simulink model "IEEE13NF_unbal"  (Simulink 8.5)
settings: Solver=ode4  StartTime=0.0  StopTime=10  FixedStep=Ts  RelTol=1e-3
PreLoadFcn:
  | Ts=0.01;
PostLoadFcn:
  | Ts=0.01;
InitFcn:
  | Ts=0.01;
StartFcn:
  | Ts=0.01;
libraries: dspindex x6, opal_lib x2, rtlab x2, rtlab_phasor x1
settings Model: Creator=ZhiqiZhao  LastModifiedBy=Jaimie.Swartz
settings DebuggingCC: SolverPrmCheckMsg=warning  FcnCallInpInsideContextMsg=EnableAllAsWarning

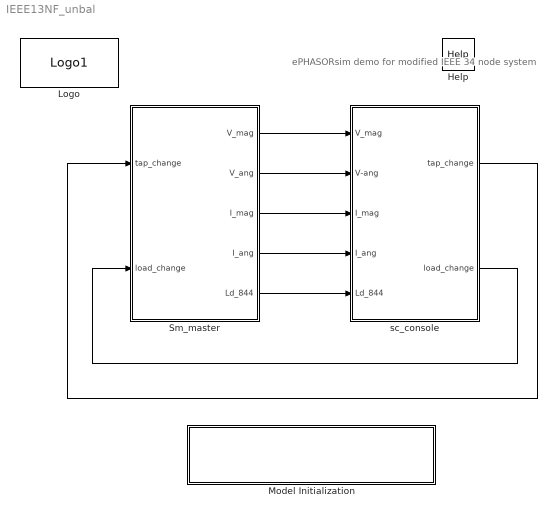
== system IEEE13NF_unbal ==
  note: ePHASORsim demo for
      | modified IEEE 34 node system
  Help : opal_lib/Help  docfile=../help/ePH_IEEE34.html
  Logo : opal_lib/Logo1  vide=[]
  Model Initialization : Subsystem  mask(Model Functions){InitFcnX=Ts=0.01;, prel=on, posl=on, inif=on, strf=on}
      mask prompts: InitFcnX "Initialisation"; prel "Preload Function"; posl "PostLoad Function"; inif "InitFcn"; strf "StartFcn"
      mask init:
      | currentBlock = gcb;
      | root = bdroot(currentBlock);
      | 
      | if ~strcmp(get_param(root,'BlockDiagramType'),'library')
      |     if prel==1
      |         set_param(root, 'PreLoadFcn', InitFcnX);
      |     else
      |         set_param(root, 'PreLoadFcn', '');
      |     end
      |     if inif==1
      |         set_param(root, 'InitFcn', InitFcnX);
      |     else
      |         set_param(root, 'InitFcn', '');
      |     end
      |     if strf==1
      |         set_param(root, 'StartFcn', InitFcnX);
      |     else
      |         set_param(root, 'StartFcn', '');
      |     end
      |     if posl==1
      |         set_param(root, 'PostLoadFcn', InitFcnX);
      |     else
      |         set_param(root, 'PostLoadFcn', '');
      |     end
      | end
      | 
      | pos = get_param(currentBlock, 'Position');
      | width = pos(3) - pos(1); height = pos(4) - pos(2);
      | txt = [ upper(root) '\n' '- InitFcn. . . . . '  get_param(root, 'InitFcn') ];
      settings: CopyFcn=set_param(gcb,'LinkStatus','none')
      mask Display: text(5, height*0.5, txt, 'horizontalAlignment', 'left', 'verticalAlignment', 'middle') ;
  Sm_master : Subsystem
  sc_console : Subsystem
  wires:
  Sm_master/1(V_mag) -> sc_console/1(V_mag)
  Sm_master/2(V_ang) -> sc_console/2(V-ang)
  Sm_master/5(Ld_844) -> sc_console/5(Ld_844)
  sc_console/1(tap_change) -> Sm_master/1(tap_change)
  sc_console/2(load_change) -> Sm_master/2(load_change)
  Sm_master/3(I_mag) -> sc_console/3(I_mag)
  Sm_master/4(I_ang) -> sc_console/4(I_ang)

== system IEEE13NF_unbal/Model Initialization ==

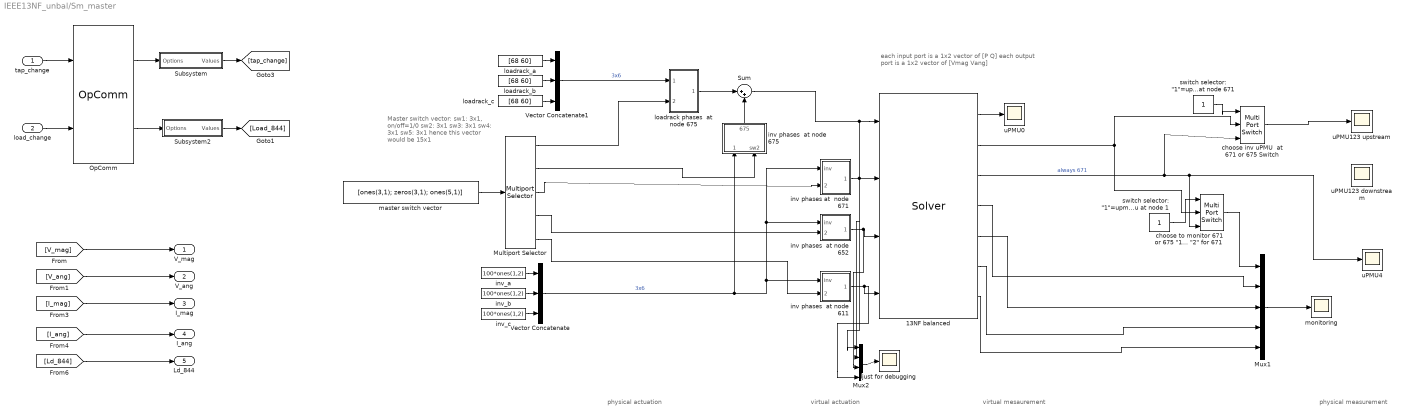
== system IEEE13NF_unbal/Sm_master ==
  note: Master switch vector:
      | sw1: 3x1, on/off=1/0
      | sw2: 3x1
      | sw3: 3x1
      | sw4: 3x1
      | sw5: 3x1
      | hence this vector would be 15x1
  note: virtual actuation
  note: virtual mesaurement
  note: physical measurement
  note: physical actuation
  note: each input port is a 1x2 vector of [P Q]
      | each output port is a 1x2 vector of [Vmag Vang]
  tap_change : Inport
  load_change : Inport  Port=2
  13NF balanced : rtlab_phasor/Solver  epname=System  extension=Excel  xls='IEEE13NF_unbal.xls'  raw='4992b.raw'  dyr='4992b.dyr'  cyme='ieee13.sxst'  powerfactory='network.dgs'  builtin=on  cyme_pf=''  cyme_unbalanced=on  lazy_netlist=on  capidir='CAPI'  fmudir='FMU'  capiprefix=capicomp_  fmuprefix=fmucomp_  logging=off  sim_mode=Dynamic simulation only (without power-flow)  pf_max_it=100  pf_tol_v=0.00000001  pf_flat_start=off  pf_smart_start=off  pf_export=on  np=1  exporty=off  dt=Ts  optim_threads=off  perflog_on=off  script_activate_postinit=off  script_postinit_name='python_integration_13NFunbal.py'
  Multiport Selector : dspindex/Multiport Selector  rowsOrCols=Rows  idxCellArray={ [1:3], [4:6], [7:9], 10,11 }  idxErrMode=Clip Index
  Mux1 : Mux  Inputs=5
  Mux2 : Mux
  OpComm : rtlab/OpComm  nbport=2  groupe_acq=1  subsys_rate=0  st=0  Synchronization=on  Interpolation=on  Threshold=1.0  Missed_Data=off  Sim_Time=off  Samples=off  dynSigOut=off  from_console=1  warning_done=off  writeOpCommFile=off  Offset=off
  Subsystem : Subsystem
  Subsystem2 : Subsystem
  Sum : Sum  Inputs=|++
  Vector Concatenate : Concatenate  NumInputs=3  Mode=Multidimensional array  ConcatenateDimension=2
  Vector Concatenate1 : Concatenate  NumInputs=3  Mode=Multidimensional array  ConcatenateDimension=2
  choose inv uPMU  at 671 or 675 Switch : MultiPortSwitch  Inputs=2
  "choose to monitor 671 or 675 \"1\" for 675 \"2\" for 671" : MultiPortSwitch  Inputs=2
  inv phases  at node 675 : Subsystem
  inv phases  at node 611 : Subsystem
  inv phases  at node 652 : Subsystem
  inv phases at  node 671 : Subsystem
  inv_a : Constant  Value=100*ones(1,2)
  inv_b : Constant  Value=100*ones(1,2)
  inv_c : Constant  Value=100*ones(1,2)
  just for debugging : Scope
      settings: SaveName=ScopeData30
  loadrack phases  at node 675 : Subsystem
  loadrack_a : Constant  Value=[68 60]
  loadrack_b : Constant  Value=[68 60]
  loadrack_c : Constant  Value=[68 60]
  master switch vector : Constant  Value=[ones(3,1); zeros(3,1); ones(5,1)]
  monitoring : Scope
      settings: SaveName=ScopeData31
  "switch selector: \"1\"=upmu at node 675 \"2\"=upmu at node 1" : Constant
  "switch selector: \"1\"=upmu at node 675 \"2\"=upmu at node 671" : Constant
  uPMU0 : Scope
  uPMU123 downstream : Scope
      settings: SaveName=ScopeData32
  uPMU123 upstream : Scope
      settings: SaveName=ScopeData33
  uPMU4 : Scope
      settings: SaveName=ScopeData34
  V_mag : Outport
  V_ang : Outport  Port=2
  I_mag : Outport  Port=3
  I_ang : Outport  Port=4
  Ld_844 : Outport  Port=5
  wires:
  tap_change/1 -> OpComm/1
  load_change/1 -> OpComm/2
  [V_mag] -> V_mag/1
  [V_ang] -> V_ang/1
  [I_ang] -> I_ang/1
  [I_mag] -> I_mag/1
  [Ld_844] -> Ld_844/1
  OpComm/1 -> Subsystem/1(Options)
  OpComm/2 -> Subsystem2/1(Options)
  Subsystem/1(Values) -> [tap_change]
  Subsystem2/1(Values) -> [Load_844]
  loadrack_a/1 -> Vector Concatenate1/1
  loadrack_b/1 -> Vector Concatenate1/2
  loadrack_c/1 -> Vector Concatenate1/3
  Vector Concatenate1/1 -> loadrack phases  at node 675/1(loadrack)  "3x6"
  inv_a/1 -> Vector Concatenate/1
  inv_b/1 -> Vector Concatenate/2
  inv_c/1 -> Vector Concatenate/3
  Sum/1 -> Mux2/1, 13NF balanced/1
  Vector Concatenate/1 -> inv phases  at node 675/1(loadrack), inv phases  at node 611/1(inv), inv phases at  node 671/1(inv), inv phases  at node 652/1(inv)  "3x6"
  inv phases at  node 671/1(671) -> Mux2/2, 13NF balanced/2
  inv phases  at node 652/1(652) -> 13NF balanced/3, Mux2/3
  inv phases  at node 611/1(611) -> 13NF balanced/4, Mux2/4
  13NF balanced/7 -> Mux1/5
  13NF balanced/5 -> Mux1/3
  13NF balanced/4 -> Mux1/2
  "switch selector: \"1\"=upmu at node 675 \"2\"=upmu at node 671"/1 -> choose inv uPMU  at 671 or 675 Switch/1
  13NF balanced/1 -> uPMU0/1
  choose inv uPMU  at 671 or 675 Switch/1 -> uPMU123 upstream/1
  13NF balanced/3 -> choose inv uPMU  at 671 or 675 Switch/3, "choose to monitor 671 or 675 \"1\" for 675 \"2\" for 671"/3, uPMU4/1  "always 671"
  "choose to monitor 671 or 675 \"1\" for 675 \"2\" for 671"/1 -> Mux1/1
  13NF balanced/6 -> Mux1/4
  Mux1/1 -> monitoring/1
  ? -> uPMU123 downstream/1
  loadrack phases  at node 675/1(675) -> Sum/1
  inv phases  at node 675/1(675) -> Sum/2
  master switch vector/1 -> Multiport Selector/1
  Multiport Selector/1 -> loadrack phases  at node 675/2(sw1)
  Multiport Selector/2 -> inv phases  at node 675/2(sw2)
  Multiport Selector/3 -> inv phases at  node 671/2(sw3)
  Multiport Selector/4 -> inv phases  at node 652/2(sw4)
  Multiport Selector/5 -> inv phases  at node 611/2(sw5)
  Mux2/1 -> just for debugging/1
  "switch selector: \"1\"=upmu at node 675 \"2\"=upmu at node 1"/1 -> "choose to monitor 671 or 675 \"1\" for 675 \"2\" for 671"/1
  13NF balanced/2 -> "choose to monitor 671 or 675 \"1\" for 675 \"2\" for 671"/2, choose inv uPMU  at 671 or 675 Switch/2

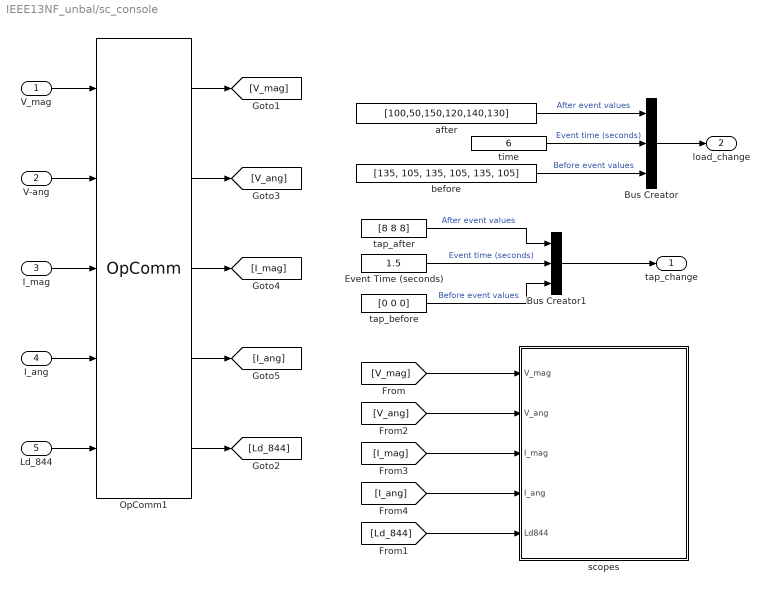
== system IEEE13NF_unbal/sc_console ==
  V_mag : Inport
  V-ang : Inport  Port=2
  I_mag : Inport  Port=3
  I_ang : Inport  Port=4
  Ld_844 : Inport  Port=5
  Bus Creator : BusCreator  Inputs=3
  Bus Creator1 : BusCreator  Inputs=3
  Event Time (seconds) : Constant  Value=1.5
  OpComm1 : rtlab/OpComm  nbport=5  groupe_acq=1  subsys_rate=0  st=0  Synchronization=on  Interpolation=on  Threshold=1.0  Missed_Data=off  Sim_Time=off  Samples=off  dynSigOut=off  from_console=0  warning_done=off  writeOpCommFile=off  Offset=off
  after : Constant  Value=[100,50,150,120,140,130]
  before : Constant  Value=[135, 105, 135, 105, 135, 105]
  scopes : Subsystem
  tap_after : Constant  Value=[8 8 8]
  tap_before : Constant  Value=[0 0 0]
  time : Constant  Value=6
  tap_change : Outport
  load_change : Outport  Port=2
  wires:
  V-ang/1 -> OpComm1/2
  V_mag/1 -> OpComm1/1
  OpComm1/1 -> [V_mag]
  OpComm1/2 -> [V_ang]
  time/1 -> Bus Creator/2  "Event time (seconds)"
  Bus Creator/1 -> load_change/1
  tap_after/1 -> Bus Creator1/1  "After event values"
  tap_before/1 -> Bus Creator1/3  "Before event values"
  Event Time (seconds)/1 -> Bus Creator1/2  "Event time (seconds)"
  Bus Creator1/1 -> tap_change/1
  after/1 -> Bus Creator/1  "After event values"
  before/1 -> Bus Creator/3  "Before event values"
  OpComm1/5 -> [Ld_844]
  Ld_844/1 -> OpComm1/5
  I_mag/1 -> OpComm1/3
  I_ang/1 -> OpComm1/4
  OpComm1/4 -> [I_ang]
  OpComm1/3 -> [I_mag]
  [V_mag] -> scopes/1(V_mag)
  [V_ang] -> scopes/2(V_ang)
  [I_mag] -> scopes/3(I_mag)
  [I_ang] -> scopes/4(I_ang)
  [Ld_844] -> scopes/5(Ld844)

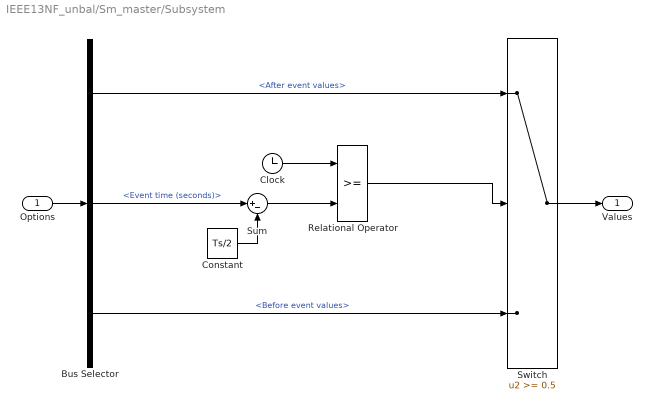
== system IEEE13NF_unbal/Sm_master/Subsystem ==
  Options : Inport
  Bus Selector : BusSelector  OutputSignals=After event values,Event time (seconds),Before event values
  Clock : Clock
  Constant : Constant  Value=Ts/2
  Relational Operator : RelationalOperator  OutDataTypeStr=boolean
  Sum : Sum  Inputs=|+-
  Switch : Switch  Threshold=0.5
  Values : Outport
  wires:
  Clock/1 -> Relational Operator/1
  Constant/1 -> Sum/2
  Sum/1 -> Relational Operator/2
  Bus Selector/2 -> Sum/1  "<Event time (seconds)>"
  Relational Operator/1 -> Switch/2
  Bus Selector/3 -> Switch/3  "<Before event values>"
  Bus Selector/1 -> Switch/1  "<After event values>"
  Switch/1 -> Values/1
  Options/1 -> Bus Selector/1

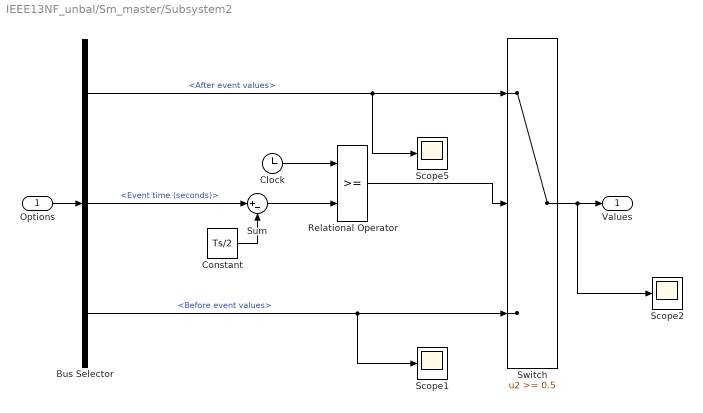
== system IEEE13NF_unbal/Sm_master/Subsystem2 ==
  Options : Inport
  Bus Selector : BusSelector  OutputSignals=After event values,Event time (seconds),Before event values
  Clock : Clock
  Constant : Constant  Value=Ts/2
  Relational Operator : RelationalOperator  OutDataTypeStr=boolean
  Scope1 : Scope
      settings: SaveName=ScopeData14
  Scope2 : Scope
      settings: SaveName=ScopeData15
  Scope5 : Scope
      settings: SaveName=ScopeData13
  Sum : Sum  Inputs=|+-
  Switch : Switch  Threshold=0.5
  Values : Outport
  wires:
  Clock/1 -> Relational Operator/1
  Constant/1 -> Sum/2
  Sum/1 -> Relational Operator/2
  Bus Selector/2 -> Sum/1  "<Event time (seconds)>"
  Relational Operator/1 -> Switch/2
  Bus Selector/3 -> Switch/3, Scope1/1  "<Before event values>"
  Bus Selector/1 -> Switch/1, Scope5/1  "<After event values>"
  Switch/1 -> Values/1, Scope2/1
  Options/1 -> Bus Selector/1

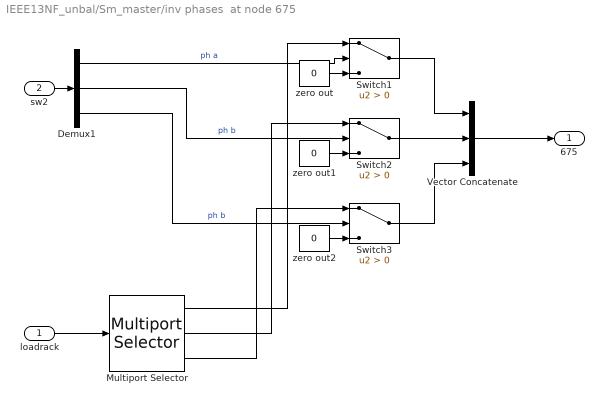
== system IEEE13NF_unbal/Sm_master/inv phases  at node 675 ==
  loadrack : Inport
  sw2 : Inport  Port=2
  Demux1 : Demux  Outputs=3
  Multiport Selector : dspindex/Multiport Selector  rowsOrCols=Columns  idxCellArray={ 1, 2, 3 }  idxErrMode=Clip Index
  Switch1 : Switch  Criteria=u2 > Threshold
  Switch2 : Switch  Criteria=u2 > Threshold
  Switch3 : Switch  Criteria=u2 > Threshold
  Vector Concatenate : Concatenate  NumInputs=3  ConcatenateDimension=2
  zero out : Constant  Value=0
  zero out1 : Constant  Value=0
  zero out2 : Constant  Value=0
  675 : Outport
  wires:
  Demux1/3 -> Switch3/2  "ph b"
  zero out2/1 -> Switch3/3
  Demux1/1 -> Switch1/2  "ph a"
  zero out/1 -> Switch1/3
  loadrack/1 -> Multiport Selector/1
  Switch2/1 -> Vector Concatenate/2
  Switch1/1 -> Vector Concatenate/1
  Switch3/1 -> Vector Concatenate/3
  Vector Concatenate/1 -> 675/1
  Multiport Selector/2 -> Switch2/1
  Multiport Selector/1 -> Switch1/1
  Multiport Selector/3 -> Switch3/1
  Demux1/2 -> Switch2/2  "ph b"
  zero out1/1 -> Switch2/3
  sw2/1 -> Demux1/1

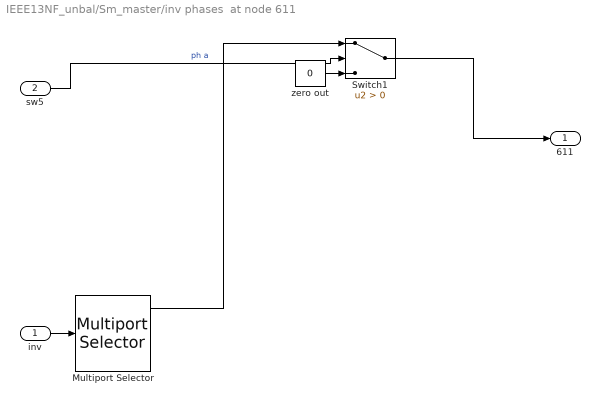
== system IEEE13NF_unbal/Sm_master/inv phases  at node 611 ==
  inv : Inport
  sw5 : Inport  Port=2
  Multiport Selector : dspindex/Multiport Selector  rowsOrCols=Columns  idxCellArray={ 1, 2, 3 }  idxErrMode=Clip Index
  Switch1 : Switch  Criteria=u2 > Threshold
  zero out : Constant  Value=0
  611 : Outport
  wires:
  sw5/1 -> Switch1/2  "ph a"
  zero out/1 -> Switch1/3
  Switch1/1 -> 611/1
  inv/1 -> Multiport Selector/1
  Multiport Selector/1 -> Switch1/1

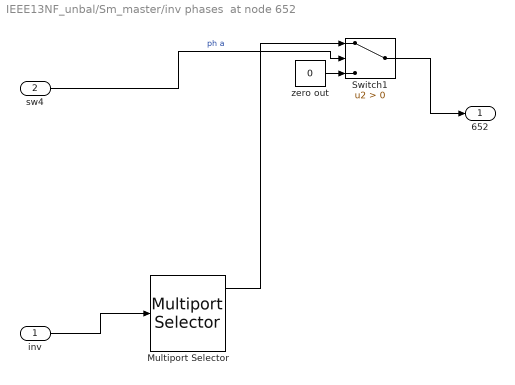
== system IEEE13NF_unbal/Sm_master/inv phases  at node 652 ==
  inv : Inport
  sw4 : Inport  Port=2
  Multiport Selector : dspindex/Multiport Selector  rowsOrCols=Columns  idxCellArray={ 1, 2, 3 }  idxErrMode=Clip Index
  Switch1 : Switch  Criteria=u2 > Threshold
  zero out : Constant  Value=0
  652 : Outport
  wires:
  sw4/1 -> Switch1/2  "ph a"
  zero out/1 -> Switch1/3
  Switch1/1 -> 652/1
  inv/1 -> Multiport Selector/1
  Multiport Selector/1 -> Switch1/1

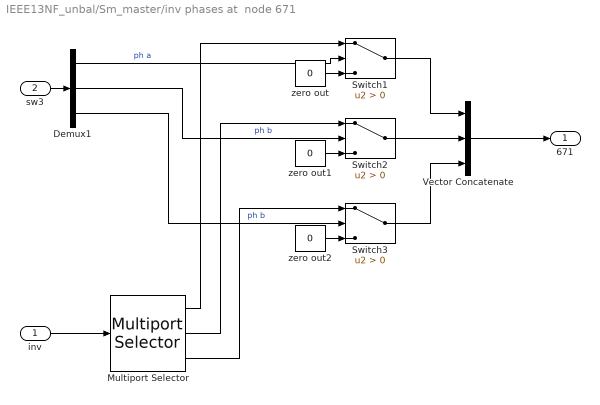
== system IEEE13NF_unbal/Sm_master/inv phases at  node 671 ==
  inv : Inport
  sw3 : Inport  Port=2
  Demux1 : Demux  Outputs=3
  Multiport Selector : dspindex/Multiport Selector  rowsOrCols=Columns  idxCellArray={ 1, 2, 3 }  idxErrMode=Clip Index
  Switch1 : Switch  Criteria=u2 > Threshold
  Switch2 : Switch  Criteria=u2 > Threshold
  Switch3 : Switch  Criteria=u2 > Threshold
  Vector Concatenate : Concatenate  NumInputs=3  ConcatenateDimension=2
  zero out : Constant  Value=0
  zero out1 : Constant  Value=0
  zero out2 : Constant  Value=0
  671 : Outport
  wires:
  Demux1/3 -> Switch3/2  "ph b"
  zero out2/1 -> Switch3/3
  Demux1/1 -> Switch1/2  "ph a"
  zero out/1 -> Switch1/3
  inv/1 -> Multiport Selector/1
  Switch2/1 -> Vector Concatenate/2
  Switch1/1 -> Vector Concatenate/1
  Switch3/1 -> Vector Concatenate/3
  Vector Concatenate/1 -> 671/1
  Multiport Selector/2 -> Switch2/1
  Multiport Selector/1 -> Switch1/1
  Multiport Selector/3 -> Switch3/1
  Demux1/2 -> Switch2/2  "ph b"
  zero out1/1 -> Switch2/3
  sw3/1 -> Demux1/1

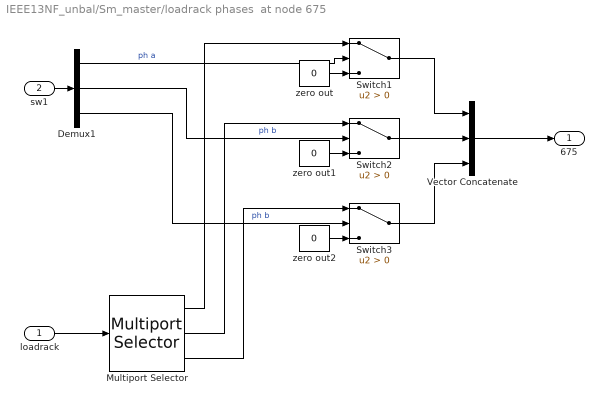
== system IEEE13NF_unbal/Sm_master/loadrack phases  at node 675 ==
  loadrack : Inport
  sw1 : Inport  Port=2
  Demux1 : Demux  Outputs=3
  Multiport Selector : dspindex/Multiport Selector  rowsOrCols=Columns  idxCellArray={ 1, 2, 3 }  idxErrMode=Clip Index
  Switch1 : Switch  Criteria=u2 > Threshold
  Switch2 : Switch  Criteria=u2 > Threshold
  Switch3 : Switch  Criteria=u2 > Threshold
  Vector Concatenate : Concatenate  NumInputs=3  ConcatenateDimension=2
  zero out : Constant  Value=0
  zero out1 : Constant  Value=0
  zero out2 : Constant  Value=0
  675 : Outport
  wires:
  Demux1/3 -> Switch3/2  "ph b"
  zero out2/1 -> Switch3/3
  Demux1/1 -> Switch1/2  "ph a"
  zero out/1 -> Switch1/3
  loadrack/1 -> Multiport Selector/1
  Switch2/1 -> Vector Concatenate/2
  Switch1/1 -> Vector Concatenate/1
  Switch3/1 -> Vector Concatenate/3
  Vector Concatenate/1 -> 675/1
  Multiport Selector/2 -> Switch2/1
  Multiport Selector/1 -> Switch1/1
  Multiport Selector/3 -> Switch3/1
  Demux1/2 -> Switch2/2  "ph b"
  zero out1/1 -> Switch2/3
  sw1/1 -> Demux1/1

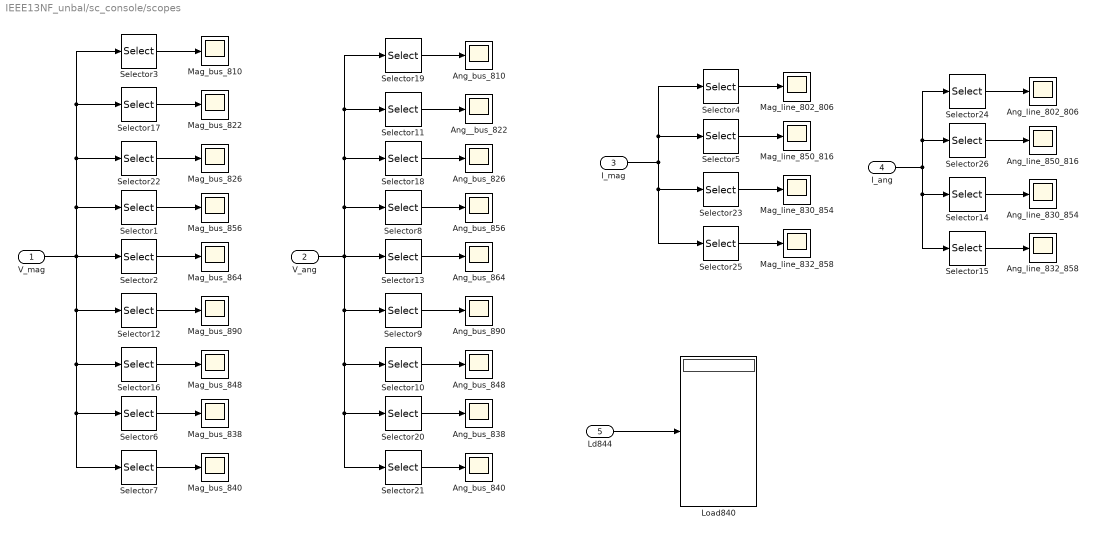
== system IEEE13NF_unbal/sc_console/scopes ==
  V_mag : Inport
  V_ang : Inport  Port=2
  I_mag : Inport  Port=3
  I_ang : Inport  Port=4
  Ld844 : Inport  Port=5
  Ang__bus_822 : Scope
      settings: YMin=0.92  YMax=1.07  SaveName=ScopeData8
  Ang_bus_{810,826,838,840,848,856,864,890} (8 alike) : Scope
      Ang_bus_810 settings: YMin=0.92  YMax=1.07  SaveName=ScopeData18
      Ang_bus_826 settings: YMin=0.92  YMax=1.07  SaveName=ScopeData9
      Ang_bus_838 settings: YMin=0.92  YMax=1.07  SaveName=ScopeData22
      Ang_bus_840 settings: YMin=0.92  YMax=1.07  SaveName=ScopeData25
      Ang_bus_848 settings: YMin=0.92  YMax=1.07  SaveName=ScopeData24
      Ang_bus_856 settings: YMin=0.92  YMax=1.07  SaveName=ScopeData10
      Ang_bus_864 settings: YMin=0.92  YMax=1.07  SaveName=ScopeData11
      Ang_bus_890 settings: YMin=0.92  YMax=1.07  SaveName=ScopeData23
  Ang_line_802_806 : Scope
      settings: YMin=0.92  YMax=1.07
  Ang_line_830_854 : Scope
      settings: YMin=0.92  YMax=1.07  SaveName=ScopeData20
  Ang_line_832_858 : Scope
      settings: YMin=0.92  YMax=1.07  SaveName=ScopeData27
  Ang_line_850_816 : Scope
      settings: YMin=0.92  YMax=1.07  SaveName=ScopeData29
  Load840 : Display
  Mag_bus_{810,822,826,838,840,848,856,864,890} (9 alike) : Scope
      Mag_bus_810 settings: YMin=0.92  YMax=1.07  SaveName=ScopeData3
      Mag_bus_822 settings: YMin=0.92  YMax=1.07  SaveName=ScopeData4
      Mag_bus_826 settings: YMin=0.92  YMax=1.07  SaveName=ScopeData5
      Mag_bus_838 settings: YMin=0.92  YMax=1.07  SaveName=ScopeData2
      Mag_bus_840 settings: YMin=0.92  YMax=1.07  SaveName=ScopeData21
      Mag_bus_848 settings: YMin=0.92  YMax=1.07  SaveName=ScopeData17
      Mag_bus_856 settings: YMin=0.92  YMax=1.07  SaveName=ScopeData6
      Mag_bus_864 settings: YMin=0.92  YMax=1.07  SaveName=ScopeData7
      Mag_bus_890 settings: YMin=0.92  YMax=1.07  SaveName=ScopeData16
  Mag_line_802_806 : Scope
      settings: YMin=0.92  YMax=1.07  SaveName=ScopeData12
  Mag_line_830_854 : Scope
      settings: YMin=0.92  YMax=1.07  SaveName=ScopeData26
  Mag_line_832_858 : Scope
      settings: YMin=0.92  YMax=1.07  SaveName=ScopeData28
  Mag_line_850_816 : Scope
      settings: YMin=0.92  YMax=1.07  SaveName=ScopeData19
  Selector1 : Selector  InputPortWidth=15  Indices=[4]
  Selector10 : Selector  InputPortWidth=15  Indices=[9 10 11]
  Selector11 : Selector  InputPortWidth=15  Indices=[2]
  Selector12 : Selector  InputPortWidth=15  Indices=[6 7 8]
  Selector13 : Selector  InputPortWidth=15  Indices=[5]
  Selector14 : Selector  InputPortWidth=12  Indices=[7 8 9]
  Selector15 : Selector  InputPortWidth=12  Indices=[10 11 12]
  Selector16 : Selector  InputPortWidth=15  Indices=[9 10 11]
  Selector17 : Selector  InputPortWidth=15  Indices=[2]
  Selector18 : Selector  InputPortWidth=15  Indices=[3]
  Selector19 : Selector  InputPortWidth=15  Indices=[1]
  Selector2 : Selector  InputPortWidth=15  Indices=[5]
  Selector20 : Selector  InputPortWidth=15  Indices=[12]
  Selector21 : Selector  InputPortWidth=15  Indices=[13 14 15]
  Selector22 : Selector  InputPortWidth=15  Indices=[3]
  Selector23 : Selector  InputPortWidth=12  Indices=[7 8 9]
  Selector24 : Selector  InputPortWidth=12  Indices=[1 2 3]
  Selector25 : Selector  InputPortWidth=12  Indices=[10 11 12]
  Selector26 : Selector  InputPortWidth=12  Indices=[4 5 6]
  Selector3 : Selector  InputPortWidth=15  Indices=[1]
  Selector4 : Selector  InputPortWidth=12  Indices=[1 2 3]
  Selector5 : Selector  InputPortWidth=12  Indices=[4 5 6]
  Selector6 : Selector  InputPortWidth=15  Indices=[12]
  Selector7 : Selector  InputPortWidth=15  Indices=[13 14 15]
  Selector8 : Selector  InputPortWidth=15  Indices=[4]
  Selector9 : Selector  InputPortWidth=15  Indices=[6 7 8]
  wires:
  Selector17/1 -> Mag_bus_822/1
  Selector22/1 -> Mag_bus_826/1
  Selector1/1 -> Mag_bus_856/1
  Selector2/1 -> Mag_bus_864/1
  Ld844/1 -> Load840/1
  Selector4/1 -> Mag_line_802_806/1
  Selector3/1 -> Mag_bus_810/1
  Selector5/1 -> Mag_line_850_816/1
  Selector12/1 -> Mag_bus_890/1
  Selector16/1 -> Mag_bus_848/1
  Selector6/1 -> Mag_bus_838/1
  Selector7/1 -> Mag_bus_840/1
  V_mag/1 -> Selector7/1, Selector6/1, Selector16/1, Selector12/1, Selector3/1, Selector17/1, Selector22/1, Selector1/1, Selector2/1
  V_ang/1 -> Selector21/1, Selector20/1, Selector10/1, Selector9/1, Selector19/1, Selector11/1, Selector18/1, Selector8/1, Selector13/1
  Selector23/1 -> Mag_line_830_854/1
  I_ang/1 -> Selector14/1, Selector15/1, Selector26/1, Selector24/1
  Selector25/1 -> Mag_line_832_858/1
  I_mag/1 -> Selector5/1, Selector4/1, Selector23/1, Selector25/1
  Selector24/1 -> Ang_line_802_806/1
  Selector26/1 -> Ang_line_850_816/1
  Selector14/1 -> Ang_line_830_854/1
  Selector15/1 -> Ang_line_832_858/1
  Selector21/1 -> Ang_bus_840/1
  Selector19/1 -> Ang_bus_810/1
  Selector11/1 -> Ang__bus_822/1
  Selector18/1 -> Ang_bus_826/1
  Selector8/1 -> Ang_bus_856/1
  Selector13/1 -> Ang_bus_864/1
  Selector9/1 -> Ang_bus_890/1
  Selector10/1 -> Ang_bus_848/1
  Selector20/1 -> Ang_bus_838/1
